simulink model "feedback_plant"  (R2020b)
settings: Solver=FixedStepDiscrete  StartTime=0.0  StopTime=10.0  FixedStep=1e-6  MaxStep=0.1  RelTol=1e-3  EnableMultiTasking=on
settings Model: ModifiedByFormat=The MathWorks Inc.  Creator=The MathWorks, Inc.  LastModifiedBy=The MathWorks Inc.
settings SolverCC: AutoInsertRateTranBlk=on
settings DataIOCC: SaveFormat=Array  ReturnWorkspaceOutputs=off
settings OptimizationCC: DefaultParameterBehavior=Inlined  ExpressionDepthLimit=2147483647  LifeSpan=1
settings DebuggingCC: UnderspecifiedInitializationDetection=Classic  MergeDetectMultiDrivingBlocksExec=none  SolverPrmCheckMsg=warning  FcnCallInpInsideContextMsg=warning  AllowSymbolicDim=off  StateNameClashWarn=warning  SFUnexpectedBacktrackingDiag=warning  SFNoUnconditionalDefaultTransitionDiag=warning  SFExecutionAtInitializationDiag=none  ArithmeticOperatorsInVariantConditions=warning
settings HardwareCC: ProdBitPerPointer=32  ProdBitPerSizeT=32  ProdBitPerPtrDiffT=32  ProdLargestAtomicFloat=None  ProdIntDivRoundTo=Undefined  ProdEndianess=Unspecified  ProdWordSize=32  ProdHWDeviceType=32-bit Generic
settings ModelReferenceCC: PropagateSignalLabelsOutOfModel=off
settings SFSimCC: SimUseLocalCustomCode=off  CustomCodeUndefinedFunction=UseInterfaceOnly
settings RTWCC: RTWUseLocalCustomCode=off
settings CodeAppCC: StateflowObjectComments=on
settings GRTTargetCC: TargetLangStandard=C89/C90 (ANSI)  CombineOutputUpdateFcns=off  GRTInterface=on
settings ConfigComp: CovMetricSettings=dw  CovSaveCumulativeToWorkspaceVar=on  CovSaveSingleToWorkspaceVar=on  CovExternalEMLEnable=off  CovSFcnEnable=off

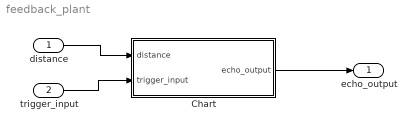
== system feedback_plant ==
  distance : Inport  OutDataTypeStr=double
  trigger_input : Inport  Port=2  OutDataTypeStr=uint8
  Chart : Stateflow chart  TreatAsAtomicUnit=on
  echo_output : Outport  OutDataTypeStr=uint8
  wires:
  distance/1 -> Chart/1(distance)
  Chart/1(echo_output) -> echo_output/1
  trigger_input/1 -> Chart/2(trigger_input)

== stateflow chart feedback_plant/Chart ==
  state OFF
    en:
    dist_sat = distance;
    if (distance <= 2)
    dist_sat = double(2);
    end
    if (distance >= 400)
    dist_sat = double(400);
    end
    counter_trig=0;
    echo_output=0;
  state ON
    en, du:
    counter_trig= counter_trig +1;
  state ON1
    en:
    echo_output=1;
  (default) -> OFF
  (junction 15) -> OFF
  (junction 14) -> (junction 15)
  OFF -> ON : [trigger_input==1]
  ON -> (junction 9) : [trigger_input==0]
  (junction 9) -> (junction 14) [order 2]
  (junction 9) -> ON1 [order 1] : [counter_trig>=10]
  (junction 21) -> (junction 14)
  ON1 -> (junction 21) : after(dist_sat*58, usec)
  data: distance input double; echo_output output uint8; trigger_input input uint8; counter_trig local uint8; dist_sat local double
